simulink model "assignment3_1"  (R2016a)
settings: Solver=VariableStepAuto  StartTime=0.0  StopTime=500  RelTol=1e-3
values from neighbouring files (symbols this model uses):
  A = [ -0.005131  0        0       0       0 ... (first row only)    [assgt3_1.m]
  B = [ -0.629  0.624 ... (first row only)    [assgt3_1.m]
  Bd = [ -0.062 -0.067 ... (first row only)    [assgt3_1.m]
  C = [ -0.7223 -0.5170  0.3386 -0.1633  0.1121 ... (first row only)    [assgt3_1.m]
  Vvar = kv*ones(2,1)    [assgt3_1.m]
  Wvar = kw*ones(2,1)    [assgt3_1.m]
  y1amp = 1    [assgt3_1.m]
  y1freq = 0.005    [assgt3_1.m]
  y2amp = 0    [assgt3_1.m]
  y2freq = 0.005    [assgt3_1.m]
undefined symbols (not defined in the file or in its folder): KFL, lqrK
settings Model: Creator=Sondre  LastModifiedBy=Sondre

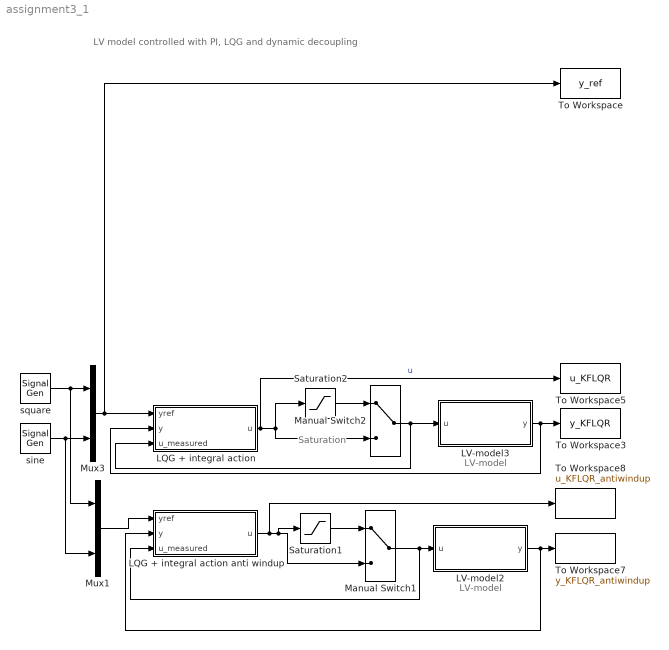
== system assignment3_1 ==
  note: Saturation
  note: LV-model
  note: LV model controlled with PI, LQG and dynamic decoupling
  note: LV-model
  LQG + integral action : Subsystem
  LQG + integral action anti windup : Subsystem
  LV-model2 : Subsystem
  LV-model3 : Subsystem
  Manual Switch1 : ManualSwitch
  Manual Switch2 : ManualSwitch
  Mux1 : Mux  Inputs=2
  Mux3 : Mux  Inputs=2
  Saturation1 : Saturate
  Saturation2 : Saturate
  To Workspace : ToWorkspace  VariableName=y_ref  SaveFormat=Structure With Time  SampleTime=-1
  To Workspace3 : ToWorkspace  VariableName=y_KFLQR  SaveFormat=Structure With Time  SampleTime=-1
  To Workspace5 : ToWorkspace  VariableName=u_KFLQR  SaveFormat=Structure With Time  SampleTime=-1
  To Workspace7 : ToWorkspace  VariableName=y_KFLQR_antiwindup  SaveFormat=Structure With Time  SampleTime=-1
  To Workspace8 : ToWorkspace  VariableName=u_KFLQR_antiwindup  SaveFormat=Structure With Time  SampleTime=-1
  sine : SignalGenerator  Amplitude=y2amp  Frequency=y2freq
  square : SignalGenerator  WaveForm=square  Amplitude=y1amp  Frequency=y1freq
  wires:
  square/1 -> Mux3/1, Mux1/1
  sine/1 -> Mux3/2, Mux1/2
  Mux3/1 -> To Workspace/1, LQG + integral action/1(yref)
  Manual Switch2/1 -> LQG + integral action/3(u_measured), LV-model3/1(u)
  Saturation2/1 -> Manual Switch2/1
  LQG + integral action/1(u) -> Manual Switch2/2, Saturation2/1, To Workspace5/1  "u"
  LV-model3/1(y) -> To Workspace3/1, LQG + integral action/2(y)
  Saturation1/1 -> Manual Switch1/1
  LQG + integral action anti windup/1(u) -> Manual Switch1/2, Saturation1/1, To Workspace8/1
  LV-model2/1(y) -> LQG + integral action anti windup/2(y), To Workspace7/1
  Manual Switch1/1 -> LQG + integral action anti windup/3(u_measured), LV-model2/1(u)
  Mux1/1 -> LQG + integral action anti windup/1(yref)

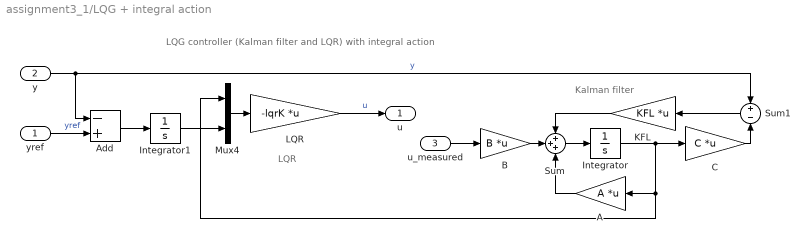
== system assignment3_1/LQG + integral action ==
  note: LQG controller (Kalman filter and LQR) with integral action
  note: LQR
  note: Kalman filter
  yref : Inport
  y : Inport  Port=2
  u_measured : Inport  Port=3
  A : Gain  Gain=A  Multiplication=Matrix(K*u)
  Add : Sum  Inputs=-+
  B : Gain  Gain=B  Multiplication=Matrix(K*u)
  C : Gain  Gain=C  Multiplication=Matrix(K*u)
  Integrator : Integrator  InitialCondition=[0 0 0 0 0]
  Integrator1 : Integrator  InitialCondition=[0 0]
  KFL : Gain  Gain=KFL  Multiplication=Matrix(K*u)
  LQR : Gain  Gain=-lqrK  Multiplication=Matrix(K*u)
  Mux4 : Mux  Inputs=2
  Sum : Sum  Inputs=+++
  Sum1 : Sum  Inputs=+-
  u : Outport
  wires:
  LQR/1 -> u/1  "u"
  B/1 -> Sum/2
  KFL/1 -> Sum/1
  Sum/1 -> Integrator/1
  A/1 -> Sum/3
  Integrator/1 -> C/1, A/1, Mux4/1
  C/1 -> Sum1/2
  Sum1/1 -> KFL/1
  Mux4/1 -> LQR/1
  u_measured/1 -> B/1
  yref/1 -> Add/2  "yref"
  y/1 -> Sum1/1, Add/1  "y"
  Integrator1/1 -> Mux4/2
  Add/1 -> Integrator1/1

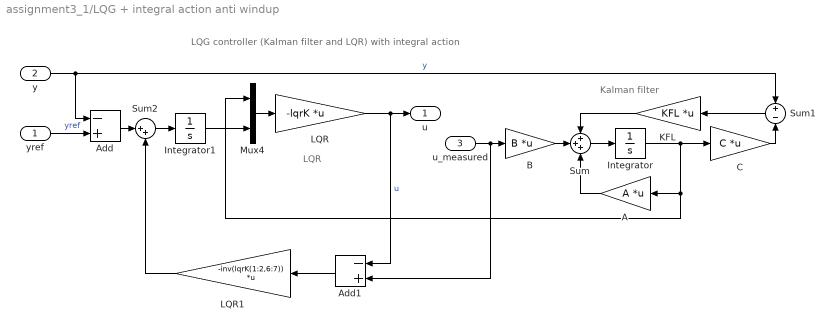
== system assignment3_1/LQG + integral action anti windup ==
  note: LQG controller (Kalman filter and LQR) with integral action
  note: LQR
  note: Kalman filter
  yref : Inport
  y : Inport  Port=2
  u_measured : Inport  Port=3
  A : Gain  Gain=A  Multiplication=Matrix(K*u)
  Add : Sum  Inputs=-+
  Add1 : Sum  Inputs=-+
  B : Gain  Gain=B  Multiplication=Matrix(K*u)
  C : Gain  Gain=C  Multiplication=Matrix(K*u)
  Integrator : Integrator  InitialCondition=[0 0 0 0 0]
  Integrator1 : Integrator  InitialCondition=[0 0]
  KFL : Gain  Gain=KFL  Multiplication=Matrix(K*u)
  LQR : Gain  Gain=-lqrK  Multiplication=Matrix(K*u)
  LQR1 : Gain  Gain=-inv(lqrK(1:2,6:7))  Multiplication=Matrix(K*u)
  Mux4 : Mux  Inputs=2
  Sum : Sum  Inputs=+++
  Sum1 : Sum  Inputs=+-
  Sum2 : Sum  Inputs=|++
  u : Outport
  wires:
  LQR/1 -> Add1/1, u/1  "u"
  B/1 -> Sum/2
  KFL/1 -> Sum/1
  Sum/1 -> Integrator/1
  A/1 -> Sum/3
  Integrator/1 -> C/1, A/1, Mux4/1
  C/1 -> Sum1/2
  Sum1/1 -> KFL/1
  Mux4/1 -> LQR/1
  u_measured/1 -> Add1/2, B/1
  yref/1 -> Add/2  "yref"
  y/1 -> Sum1/1, Add/1  "y"
  Integrator1/1 -> Mux4/2
  Add1/1 -> LQR1/1
  Add/1 -> Sum2/1
  Sum2/1 -> Integrator1/1
  LQR1/1 -> Sum2/2

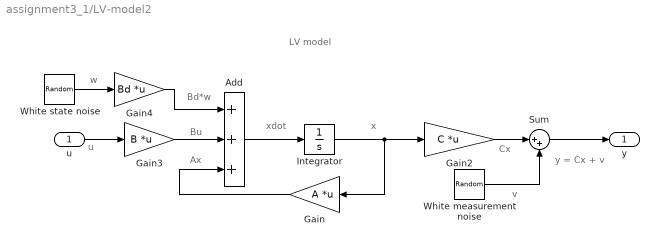
== system assignment3_1/LV-model2 ==
  note: v
  note: w
  note: y = Cx + v
  note: Ax
  note: u
  note: x
  note: xdot
  note: Bd*w
  note: Bu
  note: Cx
  note: LV model
  u : Inport
  Add : Sum  Inputs=+++
  Gain : Gain  Gain=A  Multiplication=Matrix(K*u)
  Gain2 : Gain  Gain=C  Multiplication=Matrix(K*u)
  Gain3 : Gain  Gain=B  Multiplication=Matrix(K*u)
  Gain4 : Gain  Gain=Bd  Multiplication=Matrix(K*u)
  Integrator : Integrator
  Sum : Sum  Inputs=|++
  White measurement noise : RandomNumber  Variance=Vvar  Seed=[3 4]  SampleTime=0
  White state noise : RandomNumber  Variance=Wvar  Seed=[1 2]  SampleTime=0
  y : Outport
  wires:
  u/1 -> Gain3/1
  White measurement noise/1 -> Sum/2
  Sum/1 -> y/1
  Gain2/1 -> Sum/1
  White state noise/1 -> Gain4/1
  Add/1 -> Integrator/1
  Gain/1 -> Add/3
  Gain3/1 -> Add/2
  Integrator/1 -> Gain2/1, Gain/1
  Gain4/1 -> Add/1

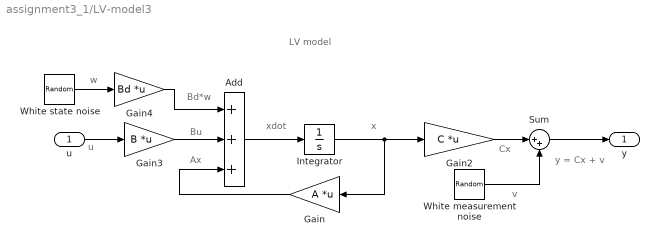
== system assignment3_1/LV-model3 ==
  note: v
  note: w
  note: y = Cx + v
  note: Ax
  note: u
  note: x
  note: xdot
  note: Bd*w
  note: Bu
  note: Cx
  note: LV model
  u : Inport
  Add : Sum  Inputs=+++
  Gain : Gain  Gain=A  Multiplication=Matrix(K*u)
  Gain2 : Gain  Gain=C  Multiplication=Matrix(K*u)
  Gain3 : Gain  Gain=B  Multiplication=Matrix(K*u)
  Gain4 : Gain  Gain=Bd  Multiplication=Matrix(K*u)
  Integrator : Integrator
  Sum : Sum  Inputs=|++
  White measurement noise : RandomNumber  Variance=Vvar  Seed=[3 4]  SampleTime=0
  White state noise : RandomNumber  Variance=Wvar  Seed=[1 2]  SampleTime=0
  y : Outport
  wires:
  u/1 -> Gain3/1
  White measurement noise/1 -> Sum/2
  Sum/1 -> y/1
  Gain2/1 -> Sum/1
  White state noise/1 -> Gain4/1
  Add/1 -> Integrator/1
  Gain/1 -> Add/3
  Gain3/1 -> Add/2
  Integrator/1 -> Gain2/1, Gain/1
  Gain4/1 -> Add/1
